simulink model "sensor_estimator"  (R2020b)
settings: Solver=VariableStepAuto  StartTime=0.0  StopTime=10.0  RelTol=1e-3
values from neighbouring files (symbols this model uses):
  ESTIMATOR_TRANSFER_FUNCTION_DENOMINATOR = [ESTIMATOR_TIME_CONSTANT 1]    [Workshop_MATLAB.m]
  ESTIMATOR_TRANSFER_FUNCTION_NUMERATOR = [1 0]    [Workshop_MATLAB.m]
  MEASUREMENT_DELAY = 0.8    [Workshop_MATLAB.m]
  MEASUREMENT_NOISE_VARIANCE = 10^(-9)    (= 1e-09)    [Workshop_MATLAB.m]
settings Model: Creator=WLCG  LastModifiedBy=WLCG

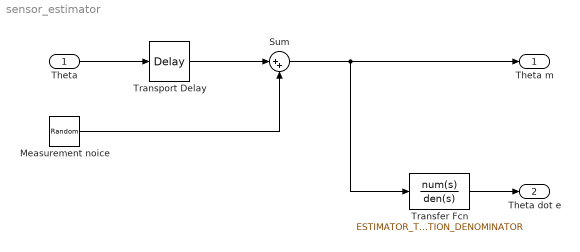
== system sensor_estimator ==
  Theta : Inport
  Measurement noice : RandomNumber  Variance=MEASUREMENT_NOISE_VARIANCE  SampleTime=0.1
  Sum : Sum  Inputs=|++
  Transfer Fcn : TransferFcn  Numerator=ESTIMATOR_TRANSFER_FUNCTION_NUMERATOR  Denominator=ESTIMATOR_TRANSFER_FUNCTION_DENOMINATOR
  Transport Delay : TransportDelay  DelayTime=MEASUREMENT_DELAY
  Theta m : Outport
  Theta dot e : Outport  Port=2
  wires:
  Transfer Fcn/1 -> Theta dot e/1
  Theta/1 -> Transport Delay/1
  Transport Delay/1 -> Sum/1
  Measurement noice/1 -> Sum/2
  Sum/1 -> Transfer Fcn/1, Theta m/1
